simulink library "scarsLibrary"  (R2019b)
settings: Solver=VariableStepAuto  StartTime=0.0  StopTime=10.0  RelTol=1e-3
undefined symbols (not defined in the file): A_x, A_y, A_z, Actuators, added_noise, axis_switch, bb, C_d, decsec, decstart, delay, Detumbling, displacement, Earth, IAU, initDay, initEuler, initYear, linsys1, mag_sat, Magnetorquers, multiplied_noise, Re, rw, scars_library, st_freq, startTime, sun_position, t_power, WGS84
libraries: $bdroot x89, aerolibutil x15, sharedtransform x12, vrlib x9, simulink x6, aerolibtransform2 x2, aerolibgravity2 x2, aerolib6dof2 x2, simulink_extras x2, aerolibatmos2 x1, aerolibnav x1
(part 1 of 2)
settings Model: Creator=asmialek  LastModifiedBy=asmialek

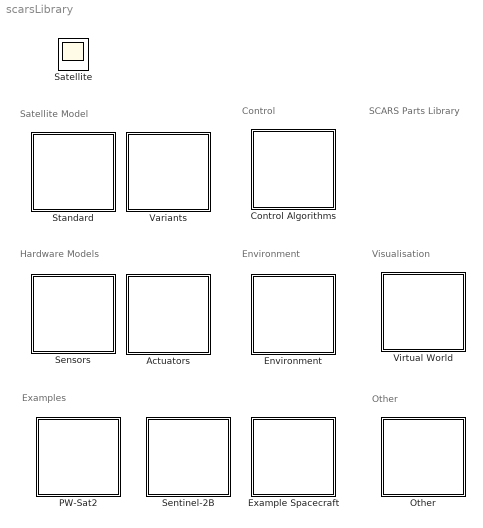
== system scarsLibrary ==
  note: SCARS
      | Parts
      | Library
  note: Environment
  note: Hardware Models
  note: Visualisation
  note: Examples
  note: Control
  note: Satellite Model
  note: Other
  " Control Algorithms " : Subsystem
  Actuators : Subsystem
  Environment : Subsystem
  Example Spacecraft : Subsystem
  Other : Subsystem
  PW-Sat2 : Subsystem
  Sensors : Subsystem
  Sentinel-2B : Subsystem
  Standard : Subsystem
  Variants : Subsystem
  Virtual World : Subsystem
  Satellite : Scope

== system scarsLibrary/ Control Algorithms  ==
  note: Control
  B-dot Algorithm : Subsystem  mask{k_gain=3e-5}
      mask prompts: k_gain "K Gain"
  LQR Controller : Subsystem  mask(Linear-Quadratic Regulator){A=linsys1.A, B=linsys1.B, Q=diag([100 100 100 1 1 1]), R=diag([ 1 1 1 ])}
      mask help: An optimal control method that uses a solution which in simplest form minimizes the quadratic cost function, based on matrices minimizing error in each state and control effor of each input, to generate static gain matrix K.
      mask init:
      | K = lqr(A, B, Q, R)
  Lat/Long to Heading : Subsystem
  PID Controller : Subsystem  mask{Kp=1, Ki=0, Kd=0, pid_sat_max=inf, pid_sat_min=-inf, pid_dz_max=0, pid_dz_min=0}
      mask prompts: Kp "Proportional Gain"; Ki "Integral Gain"; Kd "Derivative Gain"; pid_sat_max "Saturation Max Limit"; pid_sat_min "Saturation Min Limit"; pid_dz_max "Dead Zone Max Limit"; pid_dz_min "Dead Zone Min Limit"

== system scarsLibrary/Actuators ==
  note: Actuators
  Bang-Bang Thrusters : Subsystem
  Basic Thrusters : Subsystem  mask{delay=0, thrust_max=0, thrust_min=0, power=0}
      mask prompts: delay "Transport Delay"; thrust_max "Maximum Thurst"; thrust_min "Minumum Thurst"; power "Power Consumption"
  Drag Sail : Subsystem  mask{area_vector=[0.01 2 2], C_d=[1 1 1], ds_time=0, ds_duration=0, ds_moments=0}
      mask prompts: area_vector "Sail area (X, Y, Z) [m]"; C_d "Drag coefficient (X, Y, Z)"; ds_time "Deployment time [s]"; ds_duration "Deployment duration [s]"; ds_moments "Deployment moments [Nm]"
  Drag Sail (1-axis) : Subsystem  mask{sail_axis_str=X, area=0, C_d=1, deploy_time=0}
      mask prompts: sail_axis_str "Axis perpendicular to sail's plane"; area "Sail area"; C_d "Drag coefficient"; deploy_time "Deployment time"
      mask init:
      | switch sail_axis_str
      |     case 'X'
      |         A_x = area
      |         A_y = 0
      |         A_z = 0
      |     case 'Y'
      |         A_x = 0
      |         A_y = area
      |         A_z = 0
      |     case 'X'
      |         A_x = 0
      |         A_y = 0
      |         A_z = area
      | end
      mask TypeOptions sail_axis_str: X | Y | Z
  Magnetorquer (1-axis) : Subsystem  mask{mag_axis_str=X, L_mt=2.666, R_mt=3.621, l_c_mt=0.25, w_c_mt=7.965e-3, d_w_mt=4.04e-4, mag_vol_max=0, mag_vol_min=0}
      mask prompts: mag_axis_str "Operating Axis"; L_mt "L"; R_mt "R"; l_c_mt "Core Length"; w_c_mt "Core Width"; d_w_mt "Wire Diameter"; mag_vol_max "Max Voltage"; mag_vol_min "Min Voltage"
      mask init:
      | gamma_mt = 2; % empirical constant
      | 
      | mt_pre = gamma_mt*pi*l_c_mt*w_c_mt/(4*d_w_mt);
      | mt_top = (((l_c_mt/w_c_mt)^2)-1)^(3/2);
      | mt_bottom = (l_c_mt/w_c_mt)*acosh(l_c_mt/w_c_mt)-sqrt((l_c_mt/w_c_mt)-1);
      | 
      | mt_gain = mt_pre*((mt_top/mt_bottom)-1);
      | 
      | switch mag_axis_str
      |     case 'X'
      |         axis_switch = 1
      |     case 'Y'
      |         axis_switch = 2
      |     case 'Z'
      |         axis_switch = 3
      | end
      mask TypeOptions mag_axis_str: X | Y | Z
  Magnetorquers : Subsystem  mask{L_mt=2.666, R_mt=3.621, l_c_mt=0.25, w_c_mt=7.965e-3, d_w_mt=4.04e-4, mag_vol_max=3, mag_vol_min=-3}
      mask prompts: L_mt "L"; R_mt "R"; l_c_mt "Core Length"; w_c_mt "Core Width"; d_w_mt "Wire Diameter"; mag_vol_max "Max Voltage"; mag_vol_min "Min Voltage"
      mask init:
      | gamma_mt = 2; % empirical constant
      | 
      | mt_pre = gamma_mt*pi*l_c_mt*w_c_mt/(4*d_w_mt);
      | mt_top = (((l_c_mt/w_c_mt)^2)-1)^(3/2);
      | mt_bottom = (l_c_mt/w_c_mt)*acosh(l_c_mt/w_c_mt)-sqrt((l_c_mt/w_c_mt)-1);
      | 
      | mt_gain = mt_pre*((mt_top/mt_bottom)-1);
  Magnetorquers (Detumbling) : Subsystem  mask{L_mt=2.666, R_mt=3.621, l_c_mt=0.25, w_c_mt=7.965e-3, d_w_mt=4.04e-4, mag_vol_max=0, mag_vol_min=0}
      mask prompts: L_mt "L"; R_mt "R"; l_c_mt "Core Length"; w_c_mt "Core Width"; d_w_mt "Wire Diameter"; mag_vol_max "Max Voltage"; mag_vol_min "Min Voltage"
      mask init: same as scarsLibrary/Actuators/Magnetorquers
  Perfect Actuators : Subsystem  mask{k=1}
      mask prompts: k "Gain"
      mask DialogControl Control2 Prompt: (Add text here)
  Perfect Actuators (1-axis) : Subsystem  mask{axis_switch=X, k=1}
      mask prompts: axis_switch "Operating Axis"; k "Gain"
      mask TypeOptions axis_switch: X | Y | Z
      mask DialogControl Control2 Prompt: (Add text here)
  "Perfect Actuators (1-axis, vector)" : Subsystem  mask{axis_switch=X, k=1}
      mask prompts: axis_switch "Operating Axis"; k "Gain"
      mask TypeOptions axis_switch: X | Y | Z
      mask DialogControl Control2 Prompt: (Add text here)
  "Reaction Wheel (1-axis, X/Y/Z)" : Subsystem  mask{axis_switch=X, N=25e-3, R=0.1, J=1, c=0.0001, vel_max=0.0001, torq_max=0, i_max=0, rw_power=0.0001, rw_freq=0.1}
      mask prompts: axis_switch "Operating Axis"; N "Torque per unit current [Nm]"; R "Armature restitance [Ohm]"; J "Moment of inertia of wheel plus motor [kgm2]"; c "Viscous friction coefficient"; vel_max "Maximum angular velocity [rad/s]"; torq_max "Maximum torque [Nm]"; i_max "Maximum current [A]"; rw_power "Output Noise Power"; rw_freq "Noise Frequency"
      mask TypeOptions axis_switch: X | Y | Z
  "Reaction Wheel (1-axis, vector)" : Subsystem  mask(Reaction Wheel){op_vect=[1 1 1], N=(1.5e-3)/0.5, R=12, J=300e-3, c=0.0001, vel_max=6000*2*pi/60, torq_max=1.5e-3, i_max=0.5, rw_power=0.0001, rw_freq=0.1}
      mask prompts: op_vect "Operating Axis (X,Y,Z)"; N "Torque per unit current [Nm]"; R "Armature restitance [Ohm]"; J "Moment of inertia of wheel plus motor [kgm2]"; c "Viscous friction coefficient"; vel_max "Maximum angular velocity [rad/s]"; torq_max "Maximum torque [Nm]"; i_max "Maximum current [A]"; rw_power "Output Noise Power"; rw_freq "Noise Frequency"
      mask help:
      | Fast attitude control can be also achieved by the use of reaction wheels - mechanisms consisting of rotating flywheel and proportional electromagnetic torquer, such as DC motor. This allows for very precise attitude maneuvers, with the possibility to eliminate most disturbance torques.
      |
      | Inputs:
      |  Cmd - Reaction Wheel commadn voltage [V]
      |  SatStates - Bus signal from Satellite  Dynamics
      |
      | Outputs:
      |  Moment - Torque that is produced by the wheel and which acts on spacecraft (in Body frame) [Nm]
      |  WheelVel - Angular velocity of the wheel [rad/s]
      mask init:
      | op_vect = op_vect/norm(op_vect);
  Reaction Wheels : Subsystem
  Thruster : Subsystem

== system scarsLibrary/Environment ==
  Atmosphere [kg/m^3] : Subsystem
  Atmospheric Drag [N] : Subsystem
  Drag [N] : Subsystem
  Environment : Subsystem
  Gravity [N] : Subsystem  mask(Gravity){mass=0}
      mask prompts: mass "Object mass [kg]"
      mask help: Main centripetal force acting on a spacecraft on any orbit is gravity, derived from Newton's law of universal gravitation.
  Magnetic Field [nT] : Subsystem
  Sun's Position [km] : Subsystem

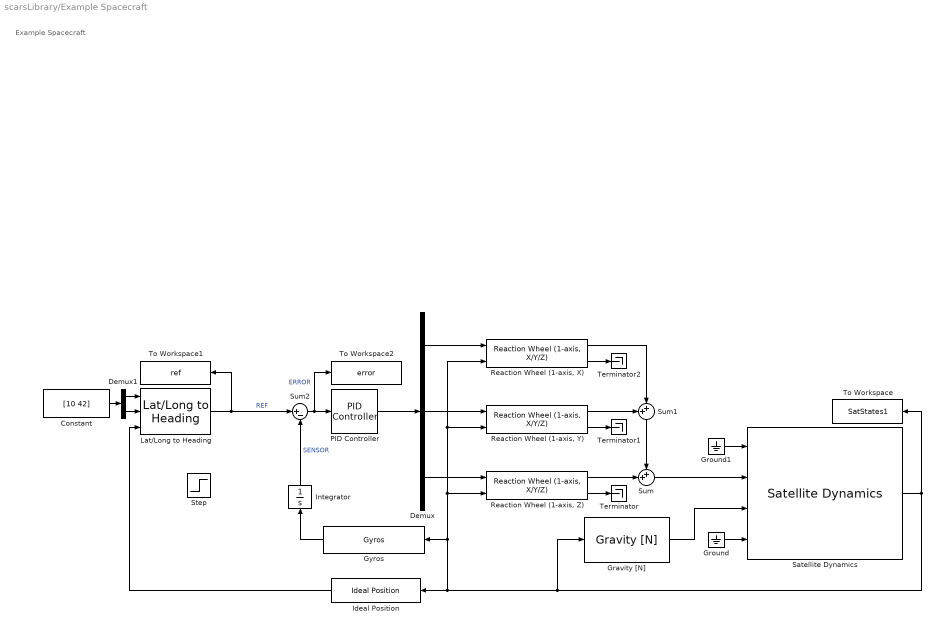
== system scarsLibrary/Example Spacecraft ==
  note: Example Spacecraft
  Constant : Constant  Value=[10 42]
  Demux : Demux  Outputs=3
  Demux1 : Demux  Outputs=2
  Gravity [N] : $bdroot/Environment/Gravity [N]  mass=1
  Ground : Ground
  Ground1 : Ground
  Gyros : $bdroot/Sensors/Gyros  g_wn=14500  g_zeta=sqrt(2)/2  g_freq=10  g_bias=0  g_power=(2*pi*0.04/360)^2  g_max=deg2rad(75)  g_min=-deg2rad(75)
  Ideal Position : $bdroot/Sensors/Ideal Position  SystemSampleTime=-1  Latency=0  AutoFrameSizeCalculation=off
  Integrator : Integrator  InitialCondition=[0.76 2.32 1.71]
  Lat/Long to Heading : $bdroot/ Control Algorithms /Lat//Long to Heading  SystemSampleTime=-1  Latency=0  AutoFrameSizeCalculation=off
  PID Controller : $bdroot/ Control Algorithms /PID Controller  Kp=700  Ki=0.01  Kd=1000  pid_sat_max=inf  pid_sat_min=-inf  pid_dz_max=0  pid_dz_min=0
  "Reaction Wheel (1-axis, X)" : $bdroot/Actuators/Reaction Wheel (1-axis, X//Y//Z)  axis_switch=X  N=(1.5e-3)/0.5  R=12  J=300e-3  c=0  vel_max=6000*2*pi/60  torq_max=1.5e-3  i_max=0.5  rw_power=0  rw_freq=0.1
  "Reaction Wheel (1-axis, Y)" : $bdroot/Actuators/Reaction Wheel (1-axis, X//Y//Z)  axis_switch=Y  N=(1.5e-3)/0.5  R=12  J=300e-3  c=0  vel_max=6000*2*pi/60  torq_max=1.5e-3  i_max=0.5  rw_power=0  rw_freq=0.1
  "Reaction Wheel (1-axis, Z)" : $bdroot/Actuators/Reaction Wheel (1-axis, X//Y//Z)  axis_switch=Z  N=(1.5e-3)/0.5  R=12  J=300e-3  c=0  vel_max=6000*2*pi/60  torq_max=1.5e-3  i_max=0.5  rw_power=0  rw_freq=0.1
  Satellite Dynamics : $bdroot/Standard/Satellite Dynamics  Parameter4=Keplerian Elements  epoch=0  mass=0  a=6356e3+400e3  e=0  incl=0  RA=0  w=0  TA=0  initEuler=[0 0 0]  initEulerRates=[0 0 0]  TA_copy=0  TA_copy_copy=400e3  TA_copy_copy_copy=[10 25]  TA_copy_copy_copy_copy=[10 25]  initEuler_copy=[0 0 0]  initEulerRates_copy=[0 0 0]
  Step : Step  Time=180  SampleTime=0
  Sum : Sum  Inputs=++|
  Sum1 : Sum  Inputs=++|
  Sum2 : Sum  Inputs=|+-
  Terminator : Terminator
  Terminator1 : Terminator
  Terminator2 : Terminator
  To Workspace : ToWorkspace  VariableName=SatStates1  SaveFormat=Timeseries  SampleTime=-1
  To Workspace1 : ToWorkspace  VariableName=ref  SaveFormat=Timeseries  SampleTime=-1
  To Workspace2 : ToWorkspace  VariableName=error  SaveFormat=Timeseries  SampleTime=-1
  wires:
  Ground/1 -> Satellite Dynamics/4
  Integrator/1 -> Sum2/2  "SENSOR"
  Demux1/1 -> Lat/Long to Heading/1
  Demux1/2 -> Lat/Long to Heading/2
  Demux/2 -> "Reaction Wheel (1-axis, Y)"/1
  PID Controller/1 -> Demux/1
  "Reaction Wheel (1-axis, Y)"/1 -> Sum1/1
  Demux/3 -> "Reaction Wheel (1-axis, Z)"/1
  "Reaction Wheel (1-axis, Y)"/2 -> Terminator1/1
  "Reaction Wheel (1-axis, X)"/1 -> Sum1/2
  "Reaction Wheel (1-axis, X)"/2 -> Terminator2/1
  "Reaction Wheel (1-axis, Z)"/2 -> Terminator/1
  Gyros/1 -> Integrator/1
  "Reaction Wheel (1-axis, Z)"/1 -> Sum/2
  Demux/1 -> "Reaction Wheel (1-axis, X)"/1
  Sum2/1 -> To Workspace2/1, PID Controller/1  "ERROR"
  Constant/1 -> Demux1/1
  Ideal Position/1 -> Lat/Long to Heading/3
  Sum1/1 -> Sum/1
  Gravity [N]/1 -> Satellite Dynamics/3
  Sum/1 -> Satellite Dynamics/2
  Ground1/1 -> Satellite Dynamics/1
  Satellite Dynamics/1 -> Ideal Position/1, Gyros/1, "Reaction Wheel (1-axis, X)"/2, "Reaction Wheel (1-axis, Y)"/2, "Reaction Wheel (1-axis, Z)"/2, Gravity [N]/1, To Workspace/1
  Lat/Long to Heading/1 -> Sum2/1, To Workspace1/1  "REF"

== system scarsLibrary/Other ==
  note: Other
  Actuator Noise : Subsystem
  Scope : Scope  NumInputPorts=2
  Subsystem : Subsystem
  Subsystem1 : Subsystem
  Subsystem4 : Subsystem
  Unit Pulse : Subsystem
  Unit Pulse Product : Subsystem
  Vector Norm : Subsystem
  "Vector Single to 3D " : Subsystem  mask{axis_switch=axis_switch}
  wires:
  Subsystem1/2(<X_ECEF>) -> Scope/2
  Subsystem1/1(<V_ECEF>) -> Scope/1

== system scarsLibrary/PW-Sat2 ==
  note: PW-Sat2
  Bus Selector : BusSelector  OutputSignals=lla,X_ECEF,V_B,A_B,Euler_B,Omega_B
  Drag Sail : Subsystem  AncestorBlock=scars_library/Actuators/Drag Sail  mask(Drag Sail){area_vector=[4 0 0], C_d=[1 0 0], ds_time=25.3*24*60*60, ds_duration=100, ds_moments=[1e-5 1e-5 1e-5]}
      mask prompts: area_vector "Sail area (X, Y, Z) [m]"; C_d "Drag coefficient (X, Y, Z)"; ds_time "Deployment time [s]"; ds_duration "Deployment duration [s]"; ds_moments "Deployment moments [Nm]"
      mask help: Drag sails use the occurrence of partial atmosphere to lower satellite's tangential velocity and therefore to quicken the deorbitation of the spacecraft. The premise is to increase area-to-mass-ratio by deploying a large and lightweight structure near the planned end-of-life of the spacecraft.
  Environment : Subsystem  AncestorBlock=scars_library/Environment/Environment  mask{area_vector=[0 0 0]}
      mask prompts: area_vector "Area Vector"
  Magnetorquers (Detumbling) : Subsystem  AncestorBlock=scars_library/Actuators/Magnetorquers (Detumbling)  mask(Magnetorquers){k_gain=-0.1, Parameter11=3, L_mt=2.666, R_mt=3.621, l_c_mt=0.25, w_c_mt=7.965e-3, d_w_mt=4.04e-4, mag_vol_max=5, Parameter9=0.2}
      mask prompts: k_gain "B-Dot algorithm gain"; Parameter11 "Maximum actuation error"; L_mt "Circuit inductance"; R_mt "Circuit resistance"; l_c_mt "Core length"; w_c_mt "Core width"; d_w_mt "Wire diameter"; mag_vol_max "Max voltage"; Parameter9 "Nominal magnetic dipole [Am^2]"
      mask help: A magnetorquer is an attitude actuator which uses Earth's geomagnetic field to generate controlling torque. The active part in the magnetorquer is the solenoid, which generates the magnetic dipole moment proportional to the current conducted by the coil.
      mask init: same as scarsLibrary/Actuators/Magnetorquers
  Satellite Dynamics : Subsystem  AncestorBlock=scars_library/Advanced/Satellite Dynamics
      mask Display: image('pw-sat-2__2.jpg'); % Use "Edit Image" on toolstrip to change.
  Scope : Scope  NumInputPorts=6
  Selector : Selector  InputPortWidth=3  IndexOptions=Index vector (dialog)  Indices=3  OutputSizes=1
  Sum : Sum  Inputs=+|+|
  To Workspace : ToWorkspace  VariableName=SatStates  SaveFormat=Timeseries  SampleTime=-1
  wires:
  Sum/1 -> Satellite Dynamics/2(M_sat)
  Bus Selector/3 -> Scope/3  "<V_B>"
  Bus Selector/6 -> Scope/6  "<Omega_B>"
  Environment/3(Moments) -> Satellite Dynamics/4(M_env)
  Satellite Dynamics/1(SatStates) -> Bus Selector/1, Magnetorquers (Detumbling)/2(SatStates), Drag Sail/1(SatStates), Environment/1(SatStates), To Workspace/1
  Bus Selector/4 -> Scope/4  "<A_B>"
  Drag Sail/2(Moment) -> Sum/1
  Bus Selector/2 -> Scope/2  "<X_ECEF>"
  Environment/1(Env) -> Drag Sail/2(Env), Magnetorquers (Detumbling)/1(Env)
  Environment/2(Forces) -> Satellite Dynamics/3(F_env)
  Drag Sail/1(Force) -> Satellite Dynamics/1(F_sat)
  Magnetorquers (Detumbling)/1(Torque) -> Sum/2
  Bus Selector/5 -> Scope/5  "<Euler_B>"
  Selector/1 -> Scope/1
  Bus Selector/1 -> Selector/1  "<lla>"

== system scarsLibrary/Sensors ==
  note: Sensors
  Accelerometer : Subsystem  mask{acc=[0 0 0], w_a=190, z_a=0.707, a_bias=[0 0 0], a_pow=0.001, a_max=inf, a_min=-inf, freq=0}
      mask prompts: acc "Sensor Location"; w_a "Natural Frequency"; z_a "Damping Ratio"; a_bias "Measurement Bias"; a_pow "Noise Power"; a_max "Upper Output Limit"; a_min "Lower Output Limit"; freq "Sampling Frequency [Hz]"
  Earth- & Sun-sensor : Subsystem
  GPS Receiver : Subsystem
  Gyros : Subsystem  mask{g_wn=1000*2*pi, g_zeta=sqrt(2)/2, g_freq=80, g_bias=0, g_power=(0.04)^2, g_max=deg2rad(100), g_min=-deg2rad(100)}
      mask prompts: g_wn "Natural Frequency [Hz]"; g_zeta "Damping Ratio"; g_freq "Operating Frequency [Hz]"; g_bias "Measurement Bias [rad/s]"; g_power "Noise Power (RND^2)"; g_max "Upper Output Limit [rad/s]"; g_min "Lower Output Limit [rad/s]"
      mask init:
      | g_wn = g_wn*2*pi;
  Ideal Angle : Subsystem
  Ideal Position : Subsystem
  Ideal Rate : Subsystem
  Magnetometer : Subsystem  mask{m_power=0.1, m_freq=10, m_bias=[0.01 0.01 0.01]}
      mask prompts: m_power "Noise Power Spectral Density"; m_freq "Sampling Frequncy [Hz]"; m_bias "Measurement Bias [nT]"
  Simple Angle : Subsystem
  Simple Position : Subsystem
  Simple Rate : Subsystem
  Star Tracker : Subsystem  mask{st_vector=[0 0 -1], st_ex_sun=20, st_ex_earth=20, st_lost=5, Parameter5=10}
      mask prompts: st_vector "Poiting Vector with respect to Body Axes"; st_ex_sun "Sun Exclusive Angle [deg]"; st_ex_earth "Earth Exclusive Angle [deg]"; st_lost "Average Lost Space Solving Time [s]"; Parameter5 "Update Rate [Hz]"

== system scarsLibrary/Sentinel-2B ==
  note: Sentinel-2B
  Actuators : Subsystem
  Environment : $bdroot/Environment/Environment  SystemSampleTime=-1  Latency=0  AutoFrameSizeCalculation=off
  OBC : Subsystem
  Satellite Dynamics : $bdroot/Standard/Satellite Dynamics  Parameter4=Keplerian Elements  epoch=0  mass=0  a=6356e3+400e3  e=0  incl=0  RA=0  w=0  TA=0  initEuler=[0 0 0]  initEulerRates=[0 0 0]  TA_copy=0  TA_copy_copy=400e3  TA_copy_copy_copy=[10 25]  TA_copy_copy_copy_copy=[10 25]  initEuler_copy=[0 0 0]  initEulerRates_copy=[0 0 0]  mask(Sattellite Dynamics){}
      mask Display: image('C:\master_thesis\scars_toolbox\resources\sentinel.jpg'); % Use "Edit Image" on toolstrip to change.
  Sensors : Subsystem
  wires:
  Sensors/1(Sensors) -> OBC/1(Sensors)
  OBC/3(MTQ) -> Actuators/4(MTQ)
  Environment/3 -> Sensors/2("Env "), Actuators/5(Env)
  Satellite Dynamics/1 -> Environment/1, Sensors/1("SatStates "), Actuators/1(SatStates)
  Actuators/2(Force) -> Satellite Dynamics/2
  Environment/1 -> Satellite Dynamics/3
  Environment/2 -> Satellite Dynamics/4
  OBC/1(RW) -> Actuators/2(RW)
  Actuators/1(Moment) -> Satellite Dynamics/1
  OBC/2(THR) -> Actuators/3(THR)

== system scarsLibrary/Standard ==
  Satellite Dynamics : Subsystem  mask(Sattellite Dynamics){Parameter4=Keplerian Elements, epoch=0, mass=0, a=6356e3+400e3, e=0, incl=0, RA=0, w=0, TA=0, initEuler=[0 0 0], initEulerRates=[0 0 0], TA_copy=0, TA_copy_copy=400e3, TA_copy_copy_copy=[10 25], TA_copy_copy_copy_copy=[10 25], initEuler_copy=[0 0 0], initEulerRates_copy=[0 0 0]}
      mask prompts: Parameter4 "Initialization method"; epoch "Epoch of ECI frame"; mass "Satellite mass [kg]"; a "Semi-major axis [m]"; e "Eccentricity"; incl "Inclination [deg]"; RA "Right ascension of the ascending node [deg]"; w "Argument of periapsis [deg]"; TA "True anomaly [deg]"; initEuler "Initial Euler orientation with reference to NED [deg]"; initEulerRates "Initial body roation rates [deg/s]"; TA_copy "True anomaly [deg]"; TA_copy_copy "Altitude [m]"; TA_copy_copy_copy "Geodetic position (latitude, longitude) [deg]"; TA_copy_copy_copy_copy "Body velocity in NED frame [m/s]"; initEuler_copy "Euler orientation with reference to NED [deg]"; initEulerRates_copy "Body roation rates [deg/s]"
      mask help: Main block of SCARS Toolbox. Allows for setting up satellite dynamics in with initial values in various coordinate system. The order of all axis, in position, velocity, orientation and rates, is always XYZ, unless otherwise stated.
      mask init:
      | Re = 6356e3;
      | G = 6.6743015e-11;
      | Re = 6356e3;
      | Me = 5.972e24;
      | 
      | if incl == 0
      |     incl = 0.00000001
      | end
      | 
      | mu = 3.986004418e14;
      | 
      | initYear = 2000;
      | initDay = 0;
      | utc = [2000 1 1 12 0 0];
      | julian = juliandate(utc);
      | juliansec = juliandate([2000 1 1 12 0 1]) - juliandate([2000 1 1 12 0 0]);
      | decstart = decyear(utc);
      | decsec = decyear(2000,1,1,12,0,1) - decyear(2000,1,1,12,0,0);
      | [r_eci, v_eci] = kep2eci(a, e, deg2rad(RA), deg2rad(incl), deg2rad(w), deg2rad(TA), mu)
      | [r_ecef,v_ecef] = eci2ecef(utc,r_eci,v_eci) % this is from aerorpace tb
      | r_lla = ecef2lla(r_ecef') % this too
      | assignin('base','R_LLA', r_lla)
      | r_lla(1:2)
      mask TypeOptions Parameter4: Keplerian Elements | ECEF Position, Velocity, Rotation | LLA Position & NED Velocity, Rotation
      mask DialogControl Container7_copy_copy Prompt: Keplerian Elements
      mask DialogControl Container7_copy Prompt: ECEF Pos, Vel, Rot
      mask DialogControl Container7 Prompt: LLA Pos & NED Vel, Rot

== system scarsLibrary/Variants ==
  Subsystem : Subsystem
  Subsystem1 : Subsystem
  Subsystem2 : Subsystem
  Subsystem3 : Subsystem

== system scarsLibrary/Virtual World ==
  note: Visualisation
  Position to VRML : Subsystem
  Quaternion to VRML : Subsystem
  SCARS VR Sink : vrlib/VR Sink  InstantiateOnLoad=on  SampleTime=-1  ViewEnable=on  RemoteChange=off  RemoteView=off  FieldsWritten=Sat.rotation.4.1.1.double#Sat.translation.3.1.1.double#Sun.translation.3.1.1.double  WorldFileName=sat_test.wrl  AutoView=off  VideoDimensions=[]  AllowVariableSize=off  FigureProperties="{'Position', 'Name', 'Viewpoint', 'CameraBound', 'CameraDirection', 'CameraPosition', 'CameraUpVector', 'ZoomFactor', 'Antialiasing', 'Headlight', 'Lighting', 'NavPanel', 'Sound', 'StatusBar', 'Stereo3D', 'Stereo3DCameraOffset', 'Stereo3DHIT', 'ToolBar', 'Textures', 'Transparency', 'Triad', 'Wireframe', 'NavZones', 'NavMode', 'NavSpeed', 'CaptureFileFormat', 'CaptureFileName', 'Record2DCompressMethod', 'Record2DCompressQuality', 'Record2D', 'Record2DFileName', 'Record2DFPS'; [5.0000000000000000e+00   9.2000000000000000e+01   5.7600000000000000e+02   3.5000000000000000e+02], '', 'Sat Cam', 'on', [0.0000000000000000e+00   0.0000000000000000e+00  -1.0000000000000000e+00], [0.0000000000000000e+00   0.0000000000000000e+00   0.0000000000000000e+00], [0.0000000000000000e+00   1.0000000000000000e+00   0.0000000000000000e+00], [1.0000000000000000e+00], 'on', 'on', 'on', 'halfbar', 'on', 'on', 'off', [1.0000000149011612e-01], [0.0000000000000000e+00], 'on', 'on', 'on', 'none', 'off', 'off', 'fly', 'normal', 'tif', '%f_anim_%n.tif', 'auto', [7.5000000000000000e+01], 'off', '%f_anim_%n.avi', 'auto'}"
      settings: SourceProductName=Simulink
  SCARS to VRML : Subsystem
  Sun's Position to ECEF : Subsystem
  wires:
  SCARS to VRML/2(Sat Pos) -> SCARS VR Sink/2
  SCARS to VRML/3(Sun Pos) -> SCARS VR Sink/3
  SCARS to VRML/1(Sat Rot) -> SCARS VR Sink/1

== system scarsLibrary/ Control Algorithms /B-dot Algorithm ==
  B : Inport
  Derivative : Derivative
  Divide : Product  Inputs=*/
  Gain2 : Gain  Gain=k_gain
  Square : Math  Operator=square  SignedPower=off  SaturateOnIntegerOverflow=on
  Vector Norm : $bdroot/Vector Norm  SystemSampleTime=-1  Latency=0  AutoFrameSizeCalculation=off
  m_ctrl : Outport
  wires:
  Derivative/1 -> Gain2/1
  Vector Norm/1 -> Square/1
  Square/1 -> Divide/2
  Divide/1 -> m_ctrl/1  "ref"
  Gain2/1 -> Divide/1
  B/1 -> Vector Norm/1, Derivative/1

== system scarsLibrary/ Control Algorithms /LQR Controller ==
  x : Inport
  Gain : Gain  Gain=-K  Multiplication=Matrix(K*u)
  u : Outport
  wires:
  x/1 -> Gain/1
  Gain/1 -> u/1

== system scarsLibrary/ Control Algorithms /Lat//Long to Heading ==
  Latitude : Inport
  Longitude : Inport  Port=2
  X_ECEF : Inport  Port=3
  Constant : Constant  Value=0
  LLA to ECEF Position : aerolibtransform2/LLA to ECEF Position  units=Metric (MKS)  ptype=Earth (WGS84)  F=1/298.257223563  R=6378137
      settings: SourceProductName=Aerospace Blockset  SourceProductBaseCode=AE
  Mux : Mux  Inputs=2
  Subsystem : $bdroot/Subsystem  SystemSampleTime=-1  Latency=0  AutoFrameSizeCalculation=off
  Sum : Sum  Inputs=-|+
  Euler_B : Outport
  wires:
  Constant/1 -> LLA to ECEF Position/2
  Latitude/1 -> Mux/1
  Longitude/1 -> Mux/2
  Mux/1 -> LLA to ECEF Position/1
  LLA to ECEF Position/1 -> Sum/1
  X_ECEF/1 -> Sum/2
  Sum/1 -> Subsystem/1
  Subsystem/1 -> Euler_B/1

== system scarsLibrary/ Control Algorithms /PID Controller ==
  Error : Inport
  Constant : Constant  Value=0
  Constant1 : Constant  Value=0
  Derivative : Derivative
  Gain : Gain  Gain=-1
  Integrator2 : Integrator  ExternalReset=either
  Kd : Gain  Gain=Kd
  Ki : Gain  Gain=Ki
  Kp : Gain  Gain=Kp
  Saturation : Saturate  UpperLimit=0.1  LowerLimit=-0.1
  Sum4 : Sum  Inputs=+++
  Switch : Switch  Criteria=u2 > Threshold  Threshold=pid_dz_max
  Switch1 : Switch  Threshold=pid_dz_max
  Switch2 : Switch  Criteria=u2 > Threshold  Threshold=-pid_dz_min
  Out : Outport
  wires:
  Integrator2/1 -> Ki/1  "theta"
  Sum4/1 -> Out/1
  Kp/1 -> Sum4/1
  Ki/1 -> Saturation/1
  Derivative/1 -> Kd/1
  Kd/1 -> Sum4/3
  Saturation/1 -> Sum4/2
  Switch1/1 -> Derivative/1, Kp/1, Integrator2/1
  Switch/1 -> Switch1/1
  Constant/1 -> Switch/3
  Constant1/1 -> Switch2/3
  Gain/1 -> Switch2/2
  Error/1 -> Integrator2/2, Switch/1, Switch/2, Gain/1, Switch2/1, Switch1/2
  Switch2/1 -> Switch1/3

== system scarsLibrary/Actuators/Bang-Bang Thrusters ==
  TorqueCmd : Inport
  Constant : Constant  Value=displacement
  Demux : Demux  Outputs=3
  Gain : Gain  Gain=-1
  Mux : Mux  Inputs=3
  Product : Product
  Thruster Pitch : Subsystem
  Thruster Roll : Subsystem
  Thruster Yaw : Subsystem
  Torque : Outport  VectorParamsAs1DForOutWhenUnconnected=off
  Moments : Outport  Port=2  VectorParamsAs1DForOutWhenUnconnected=off
  wires:
  Gain/1 -> Product/1, Torque/1
  Mux/1 -> Gain/1
  Demux/3 -> Thruster Yaw/1(Torque)
  Demux/1 -> Thruster Roll/1(Torque)
  Demux/2 -> Thruster Pitch/1(Torque)
  TorqueCmd/1 -> Demux/1
  Thruster Yaw/1(Torque Out) -> Mux/3
  Thruster Pitch/1(Torque Out) -> Mux/2
  Thruster Roll/1(Torque Out) -> Mux/1
  Constant/1 -> Product/2
  Product/1 -> Moments/1

== system scarsLibrary/Actuators/Basic Thrusters ==
  ActuatorCmd : Inport
  Abs : Abs
  Constant : Constant  Value=t_power
  Product : Product
  Saturation : Saturate  UpperLimit=thrust_max  LowerLimit=thrust_min
  Sign : Signum
  Transport Delay : TransportDelay  DelayTime=delay
  Force : Outport
  Power : Outport  Port=2
  wires:
  Abs/1 -> Saturation/1
  Sign/1 -> Product/2
  Saturation/1 -> Product/1
  Product/1 -> Force/1
  Transport Delay/1 -> Sign/1, Abs/1
  Constant/1 -> Power/1
  ActuatorCmd/1 -> Transport Delay/1

== system scarsLibrary/Actuators/Drag Sail ==
  SatStates : Inport
  Density : Inport  Port=2
  Add : Sum
  Deployment Duration : Step  Time=ds_time+ds_duration  After=-1  SampleTime=0
  Deployment Time : Step  Time=ds_time  SampleTime=0
  Depoloyment Moments : Constant  Value=ds_moments
  "Drag " : Subsystem
  Gain : Gain
  Product : Product
  Product1 : Product
  Product3 : Product
  Force : Outport
  Moment : Outport  Port=2
  wires:
  Density/1 -> "Drag "/2(Density)
  Product/1 -> Gain/1
  SatStates/1 -> "Drag "/1(SatStates)
  Deployment Time/1 -> Product1/1, Product/2
  "Drag "/1(Force) -> Product/1
  Add/1 -> Moment/1
  Depoloyment Moments/1 -> Product1/2, Product3/1
  Deployment Duration/1 -> Product3/2
  Product1/1 -> Add/1
  Product3/1 -> Add/2
  Gain/1 -> Force/1

== system scarsLibrary/Actuators/Drag Sail (1-axis) ==
  SatStates : Inport
  Bus Element In2 : Inport  Port=2  PortName=Env  Element=rho
  "Drag " : Subsystem
  Product : Product
  Step : Step  Time=5*24*60*60  SampleTime=0
  Force : Outport
  wires:
  "Drag "/1(Force) -> Product/1
  Step/1 -> Product/2
  SatStates/1 -> "Drag "/1(SatStates)
  Product/1 -> Force/1
  Bus Element In2/1 -> "Drag "/2(Density)

== system scarsLibrary/Actuators/Magnetorquer (1-axis) ==
  Voltage : Inport
  Bus Element In : Inport  Port=2  PortName=Env  Element=Magnetic Field [nT]
  Bus Element In1 : Inport  Port=3  PortName=SatStates  Element=NED2Body
  " Coil Gain" : Gain  Gain=mt_gain
  Circuit Transfer Fcn : TransferFcn  Denominator=[L_mt R_mt]
  Cross Product : vrlib/Utilities/Cross Product
      settings: SourceProductName=Simulink
  Direction Cosine Matrix to Quaternions : sharedtransform/Direction Cosine Matrix  to Quaternions  aMode=0  action=None  tolerance=eps(2)
      settings: SourceProductName=Aerospace Blockset  SourceProductBaseCode=AE
  Gain1 : Gain  Gain=1e-9
  Quaternion Rotation : aerolibutil/Quaternion Rotation
  Saturation : Saturate  UpperLimit=mag_sat  LowerLimit=-mag_sat
  "Vector Single to 3D " : $bdroot/Actuators/Vector Single to 3D   axis_switch=axis_switch
  Torque : Outport
  wires:
  Gain1/1 -> Quaternion Rotation/2
  Circuit Transfer Fcn/1 -> " Coil Gain"/1
  Saturation/1 -> Circuit Transfer Fcn/1
  Bus Element In/1 -> Gain1/1
  Quaternion Rotation/1 -> Cross Product/2
  Bus Element In1/1 -> Direction Cosine Matrix to Quaternions/1
  Direction Cosine Matrix to Quaternions/1 -> Quaternion Rotation/1
  Cross Product/1 -> Torque/1
  " Coil Gain"/1 -> "Vector Single to 3D "/1
  Voltage/1 -> Saturation/1
  "Vector Single to 3D "/1 -> Cross Product/1

== system scarsLibrary/Actuators/Magnetorquers ==
  Voltage : Inport
  Bus Element In : Inport  Port=2  PortName=Env  Element=Magnetic Field [nT]
  Bus Element In1 : Inport  Port=3  PortName=SatStates  Element=DCM_NED2B
  Cross Product : vrlib/Utilities/Cross Product
      settings: SourceProductName=Simulink
  Demux : Demux  Outputs=3
  Direction Cosine Matrix to Quaternions : sharedtransform/Direction Cosine Matrix  to Quaternions  aMode=0  action=None  tolerance=eps(2)
      settings: SourceProductName=Aerospace Blockset  SourceProductBaseCode=AE
  Gain : Gain  Gain=mt_gain
  Gain1 : Gain  Gain=1e-9
  Mux : Mux  Inputs=3
  Quaternion Rotation : aerolibutil/Quaternion Rotation
  Saturation : Saturate  UpperLimit=mag_sat  LowerLimit=-mag_sat
  Transfer Fcn : TransferFcn  Denominator=[L_mt R_mt]
  Transfer Fcn1 : TransferFcn  Denominator=[L_mt R_mt]
  Transfer Fcn2 : TransferFcn  Denominator=[L_mt R_mt]
  Moment : Outport
  wires:
  Gain1/1 -> Quaternion Rotation/2
  Mux/1 -> Gain/1
  Transfer Fcn/1 -> Mux/1
  Transfer Fcn1/1 -> Mux/3
  Transfer Fcn2/1 -> Mux/2
  Demux/1 -> Transfer Fcn/1
  Demux/2 -> Transfer Fcn2/1
  Demux/3 -> Transfer Fcn1/1
  Saturation/1 -> Demux/1
  Bus Element In/1 -> Gain1/1
  Quaternion Rotation/1 -> Cross Product/2
  Bus Element In1/1 -> Direction Cosine Matrix to Quaternions/1
  Direction Cosine Matrix to Quaternions/1 -> Quaternion Rotation/1
  Cross Product/1 -> Moment/1
  Gain/1 -> Cross Product/1
  Voltage/1 -> Saturation/1

== system scarsLibrary/Actuators/Magnetorquers (Detumbling) ==
  Bus Element In : Inport  PortName=Env  Element=Magnetic Field [nT]
  Bus Element In1 : Inport  Port=2  PortName=SatStates  Element=DCM_NED2B
  B-dot Algorithm : $bdroot/ Control Algorithms /B-dot Algorithm  k_gain=3e-5
  Cross Product : vrlib/Utilities/Cross Product
      settings: SourceProductName=Simulink
  Demux : Demux  Outputs=3
  Direction Cosine Matrix to Quaternions : sharedtransform/Direction Cosine Matrix  to Quaternions  aMode=0  action=None  tolerance=eps(2)
      settings: SourceProductName=Aerospace Blockset  SourceProductBaseCode=AE
  Gain : Gain  Gain=mt_gain
  Gain1 : Gain  Gain=1e-9
  Mux : Mux  Inputs=3
  PID Controller : $bdroot/ Control Algorithms /PID Controller  Kp=1  Ki=0  Kd=0  pid_sat_max=inf  pid_sat_min=-inf  pid_dz_max=0  pid_dz_min=0
  Quaternion Rotation : aerolibutil/Quaternion Rotation
  Saturation : Saturate  UpperLimit=mag_sat  LowerLimit=-mag_sat
  Sum : Sum  Inputs=-+|
  Transfer Fcn : TransferFcn  Denominator=[L_mt R_mt]
  Transfer Fcn1 : TransferFcn  Denominator=[L_mt R_mt]
  Transfer Fcn2 : TransferFcn  Denominator=[L_mt R_mt]
  Torque : Outport
  wires:
  PID Controller/1 -> Saturation/1
  Demux/3 -> Transfer Fcn1/1
  B-dot Algorithm/1 -> Sum/2
  Demux/1 -> Transfer Fcn/1
  Saturation/1 -> Demux/1
  Sum/1 -> PID Controller/1
  Direction Cosine Matrix to Quaternions/1 -> Quaternion Rotation/1
  Quaternion Rotation/1 -> Cross Product/2, B-dot Algorithm/1
  Mux/1 -> Gain/1
  Demux/2 -> Transfer Fcn2/1
  Transfer Fcn/1 -> Mux/1
  Bus Element In/1 -> Gain1/1
  Transfer Fcn1/1 -> Mux/3
  Cross Product/1 -> Torque/1
  Transfer Fcn2/1 -> Mux/2
  Bus Element In1/1 -> Direction Cosine Matrix to Quaternions/1
  Gain/1 -> Sum/1, Cross Product/1  "m"
  Gain1/1 -> Quaternion Rotation/2

== system scarsLibrary/Actuators/Perfect Actuators ==
  ActuatorCmd : Inport
  Demux : Demux  Outputs=3
  Gain : Gain
  Mux : Mux  Inputs=3
  Out : Outport
  wires:
  Demux/3 -> Mux/3
  Mux/1 -> Gain/1
  Demux/1 -> Mux/1
  ActuatorCmd/1 -> Demux/1
  Demux/2 -> Mux/2
  Gain/1 -> Out/1

== system scarsLibrary/Actuators/Perfect Actuators (1-axis) ==
  ActuatorCmd : Inport
  Gain : Gain
  "Vector Single to 3D  " : $bdroot/Actuators/Vector Single to 3D   axis_switch=axis_switch
  Out : Outport
  wires:
  Gain/1 -> "Vector Single to 3D  "/1
  ActuatorCmd/1 -> Gain/1
  "Vector Single to 3D  "/1 -> Out/1

== system scarsLibrary/Actuators/Perfect Actuators (1-axis, vector) ==
  ActuatorCmd : Inport
  Gain : Gain
  "Vector Single to 3D  " : $bdroot/Actuators/Vector Single to 3D   axis_switch=axis_switch
  Out : Outport
  wires:
  "Vector Single to 3D  "/1 -> Out/1
  ActuatorCmd/1 -> Gain/1
  Gain/1 -> "Vector Single to 3D  "/1

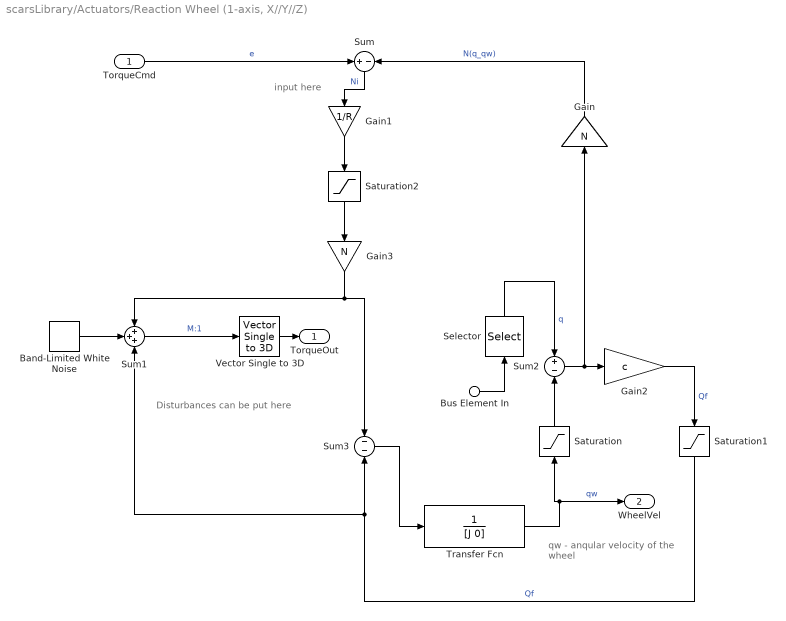
== system scarsLibrary/Actuators/Reaction Wheel (1-axis, X//Y//Z) ==
  note: qw - anqular velocity
      |  of the wheel
  note: input here
  note: Disturbances can
      | be put here
  TorqueCmd : Inport
  Bus Element In : Inport  Port=2  PortName=SatStates  Element=Omega_B
  Band-Limited White Noise : simulink/Sources/Band-Limited White Noise  Cov=rw_power  Ts=rw_freq  seed=[23341]
  Gain : Gain  Gain=N
  Gain1 : Gain  Gain=1/R
  Gain2 : Gain  Gain=c
  Gain3 : Gain  Gain=N
  Saturation : Saturate  UpperLimit=vel_max  LowerLimit=-vel_max
  Saturation1 : Saturate  UpperLimit=torq_max  LowerLimit=-torq_max
  Saturation2 : Saturate  UpperLimit=i_max  LowerLimit=-i_max
  Selector : Selector  InputPortWidth=3  IndexOptions=Index vector (dialog)  Indices=axis_switch  OutputSizes=1
  Sum : Sum  Inputs=+|-
  Sum1 : Sum  Inputs=+++
  Sum2 : Sum  Inputs=+|-
  Sum3 : Sum  Inputs=-|-
  Transfer Fcn : TransferFcn  Denominator=[J 0]
  "Vector Single to 3D " : $bdroot/Actuators/Vector Single to 3D   axis_switch=axis_switch
  TorqueOut : Outport
  WheelVel : Outport  Port=2
  wires:
  Selector/1 -> Sum2/1  "q"
  Gain/1 -> Sum/2  "N(q_qw)"
  Sum2/1 -> Gain/1, Gain2/1
  Sum1/1 -> "Vector Single to 3D "/1  "M:1"
  Saturation1/1 -> Sum1/3, Sum3/2  "Qf"
  Transfer Fcn/1 -> Saturation/1, WheelVel/1  "qw"
  Sum3/1 -> Transfer Fcn/1
  TorqueCmd/1 -> Sum/1  "e"
  Sum/1 -> Gain1/1  "Ni"
  Bus Element In/1 -> Selector/1
  "Vector Single to 3D "/1 -> TorqueOut/1
  Band-Limited White Noise/1 -> Sum1/2
  Saturation/1 -> Sum2/2
  Gain2/1 -> Saturation1/1  "Qf"
  Gain1/1 -> Saturation2/1
  Gain3/1 -> Sum1/1, Sum3/1
  Saturation2/1 -> Gain3/1

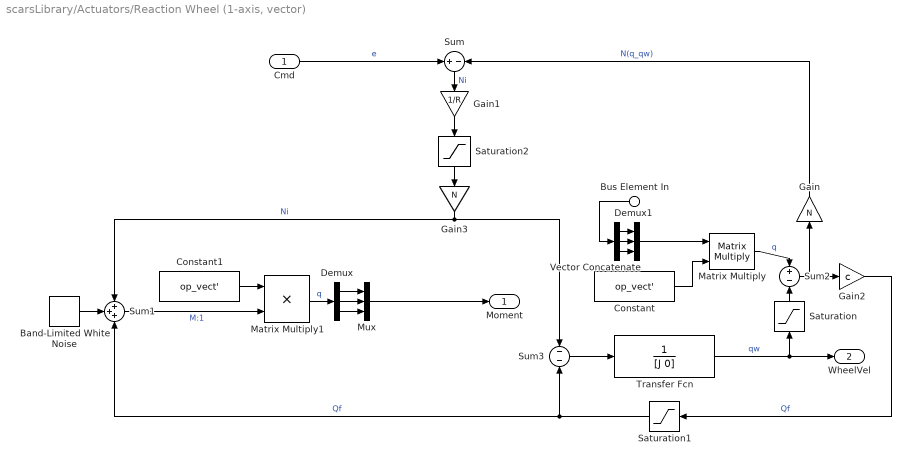
== system scarsLibrary/Actuators/Reaction Wheel (1-axis, vector) ==
  Cmd : Inport
  Bus Element In : Inport  Port=2  PortName=SatStates  Element=Omega_B
  Band-Limited White Noise : simulink/Sources/Band-Limited White Noise  Cov=rw_power  Ts=rw_freq  seed=[23341]
  Constant : Constant  Value=op_vect'  VectorParams1D=off
  Constant1 : Constant  Value=op_vect'  VectorParams1D=off
  Demux : Demux  Outputs=3
  Demux1 : Demux  Outputs=3
  Gain : Gain  Gain=N
  Gain1 : Gain  Gain=1/R
  Gain2 : Gain  Gain=c
  Gain3 : Gain  Gain=N
  Matrix Multiply : Product  Multiplication=Matrix(*)
  Matrix Multiply1 : Product
  Mux : Mux  Inputs=3
  Saturation : Saturate  UpperLimit=vel_max  LowerLimit=-vel_max
  Saturation1 : Saturate  UpperLimit=torq_max  LowerLimit=-torq_max
  Saturation2 : Saturate  UpperLimit=i_max  LowerLimit=-i_max
  Sum : Sum  Inputs=+|-
  Sum1 : Sum  Inputs=+++
  Sum2 : Sum  Inputs=+|-
  Sum3 : Sum  Inputs=-|-
  Transfer Fcn : TransferFcn  Denominator=[J 0]
  Vector Concatenate : Concatenate  NumInputs=3
  Moment : Outport
  WheelVel : Outport  Port=2
  wires:
  Gain1/1 -> Saturation2/1
  Saturation2/1 -> Gain3/1
  Sum3/1 -> Transfer Fcn/1
  Saturation1/1 -> Sum1/3, Sum3/2  "Qf"
  Transfer Fcn/1 -> Saturation/1, WheelVel/1  "qw"
  Gain/1 -> Sum/2  "N(q_qw)"
  Demux/3 -> Mux/3
  Demux/1 -> Mux/1
  Sum/1 -> Gain1/1  "Ni"
  Band-Limited White Noise/1 -> Sum1/2
  Matrix Multiply/1 -> Sum2/1  "q"
  Demux1/2 -> Vector Concatenate/2
  Vector Concatenate/1 -> Matrix Multiply/1
  Constant1/1 -> Matrix Multiply1/1
  Sum1/1 -> Matrix Multiply1/2  "M:1"
  Demux/2 -> Mux/2
  Constant/1 -> Matrix Multiply/2
  Matrix Multiply1/1 -> Demux/1  "q"
  Mux/1 -> Moment/1
  Sum2/1 -> Gain2/1, Gain/1
  Gain3/1 -> Sum3/1, Sum1/1  "Ni"
  Gain2/1 -> Saturation1/1  "Qf"
  Saturation/1 -> Sum2/2
  Demux1/3 -> Vector Concatenate/3
  Bus Element In/1 -> Demux1/1
  Cmd/1 -> Sum/1  "e"
  Demux1/1 -> Vector Concatenate/1

== system scarsLibrary/Actuators/Reaction Wheels ==
  TorqueCmd : Inport
  Bus Element In : Inport  Port=2  PortName=InBus  Element=Euler_NED
  Demux : Demux  Outputs=3
  Demux2 : Demux  Outputs=3
  Mux : Mux  Inputs=3
  Reaction Wheel Pitch : Subsystem
  Reaction Wheel Roll : Subsystem
  Reaction Wheel Yaw : Subsystem
  Torque : Outport  VectorParamsAs1DForOutWhenUnconnected=off
  wires:
  TorqueCmd/1 -> Demux/1
  Bus Element In/1 -> Demux2/1
  Reaction Wheel Yaw/1(Torque Out) -> Mux/3
  Reaction Wheel Pitch/1(Torque Out) -> Mux/2
  Demux/3 -> Reaction Wheel Yaw/2(Torque)
  Demux2/3 -> Reaction Wheel Yaw/1(Rate)
  Demux/2 -> Reaction Wheel Pitch/2(Torque)
  Demux2/2 -> Reaction Wheel Pitch/1(Rate)
  Demux2/1 -> Reaction Wheel Roll/1(Rate)
  Reaction Wheel Roll/1(Torque Out) -> Mux/1
  Demux/1 -> Reaction Wheel Roll/2(Torque)
  Mux/1 -> Torque/1

== system scarsLibrary/Actuators/Thruster ==
  ForceCmd : Inport
  Constant : Constant  Value=displacement
  Gain2 : Gain  Gain=-1
  Noise : simulink/Sources/Band-Limited White Noise  Cov=[0.1]  Ts=0.1  seed=[23341]
  Product : Product
  Relay1 : Relay  OnSwitchValue=bb.a1  OffSwitchValue=bb.a0  OnOutputValue=bb.thrust
  Relay2 : Relay  OnSwitchValue=bb.a1  OffSwitchValue=bb.a0  OnOutputValue=-bb.thrust
  Sum2 : Sum  Inputs=+++
  Transport Delay : TransportDelay  DelayTime=delay
  Force : Outport
  Moment : Outport  Port=2
  wires:
  ForceCmd/1 -> Transport Delay/1
  Relay1/1 -> Sum2/1
  Transport Delay/1 -> Gain2/1, Relay1/1
  Gain2/1 -> Relay2/1
  Noise/1 -> Sum2/2
  Sum2/1 -> Force/1
  Relay2/1 -> Product/1, Sum2/3
  Constant/1 -> Product/2
  Product/1 -> Moment/1

== system scarsLibrary/Environment/Atmosphere [kg//m^3] ==
  Bus Element In : Inport  PortName=SatStates  Element=lla
  Clock : Clock
      settings: Decimation=100
  Clock to Y/D/s : Subsystem
  "NRLMSISE-00 Atmosphere Model " : aerolibatmos2/NRLMSISE-00 Atmosphere Model  units=Metric (MKS)  lst_input=off  flux_ap_input=off  flags_input=Internal  flags=ones(1,23)  oxygen_in=off  action=Warning
      settings: SourceProductName=Aerospace Blockset  SourceProductBaseCode=AE
  "Selector " : Selector  InputPortWidth=9  IndexOptions=Index vector (dialog)  Indices=6  OutputSizes=1
  Terminator : Terminator
  Density : Outport
  wires:
  Clock to Y/D/s/1(Year) -> "NRLMSISE-00 Atmosphere Model "/2
  Clock to Y/D/s/3(sec) -> "NRLMSISE-00 Atmosphere Model "/4
  "Selector "/1 -> Density/1
  Bus Element In/1 -> "NRLMSISE-00 Atmosphere Model "/1
  Clock/1 -> Clock to Y/D/s/1(Clock)
  Clock to Y/D/s/2(Day) -> "NRLMSISE-00 Atmosphere Model "/3
  "NRLMSISE-00 Atmosphere Model "/1 -> Terminator/1
  "NRLMSISE-00 Atmosphere Model "/2 -> "Selector "/1

== system scarsLibrary/Environment/Atmospheric Drag [N] ==
  SatStates : Inport
  Atmosphere [kg/m^3] : $bdroot/Environment/Atmosphere [kg//m^3]  SystemSampleTime=-1  Latency=0  AutoFrameSizeCalculation=off
  Drag [N] : $bdroot/Environment/Drag [N]  SystemSampleTime=-1  Latency=0  AutoFrameSizeCalculation=off
  Force : Outport
  wires:
  Atmosphere [kg/m^3]/1 -> Drag [N]/2
  SatStates/1 -> Drag [N]/1, Atmosphere [kg/m^3]/1
  Drag [N]/1 -> Force/1

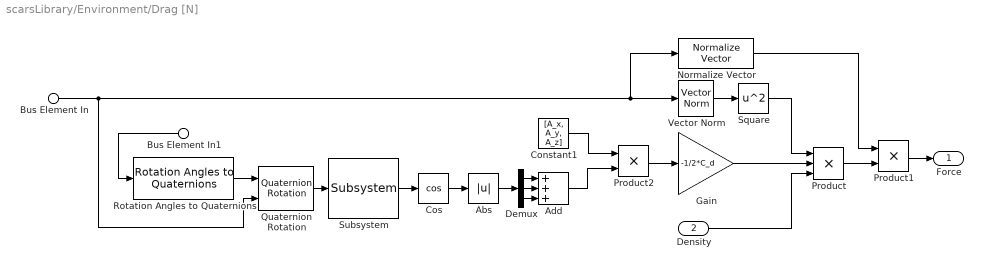
== system scarsLibrary/Environment/Drag [N] ==
  Bus Element In : Inport  PortName=SatStates  Element=V_B
  Bus Element In1 : Inport  PortName=SatStates  Element=Euler_B
  Density : Inport  Port=2
  Abs : Abs
  Add : Sum  Inputs=+++
  Constant1 : Constant  Value=[A_x, A_y, A_z]
  Cos : Trigonometry  Operator=cos
  Demux : Demux  Outputs=3
  Gain : Gain  Gain=-1/2*C_d
  Normalize Vector : vrlib/Utilities/Normalize Vector  maxzero=0
      settings: SourceProductName=Simulink
  Product : Product  Inputs=3
  Product1 : Product
  Product2 : Product
  Quaternion Rotation : aerolibutil/Quaternion Rotation
  Rotation Angles to Quaternions : sharedtransform/Rotation Angles to Quaternions  rotationOrder=XYZ  aMode=aMode
      settings: SourceProductName=Aerospace Blockset  SourceProductBaseCode=AE
  Square : Math  Operator=square  SignedPower=off  SaturateOnIntegerOverflow=on
  Subsystem : $bdroot/Subsystem  SystemSampleTime=-1  Latency=0  AutoFrameSizeCalculation=off
  Vector Norm : $bdroot/Vector Norm  SystemSampleTime=-1  Latency=0  AutoFrameSizeCalculation=off
  Force : Outport
  wires:
  Gain/1 -> Product/2
  Product/1 -> Product1/2
  Product1/1 -> Force/1
  Normalize Vector/1 -> Product1/1
  Density/1 -> Product/3
  Bus Element In1/1 -> Rotation Angles to Quaternions/1
  Constant1/1 -> Product2/1
  Product2/1 -> Gain/1
  Rotation Angles to Quaternions/1 -> Quaternion Rotation/1
  Bus Element In/1 -> Vector Norm/1, Normalize Vector/1, Quaternion Rotation/2
  Quaternion Rotation/1 -> Subsystem/1
  Subsystem/1 -> Cos/1
  Demux/1 -> Add/1
  Demux/2 -> Add/2
  Demux/3 -> Add/3
  Cos/1 -> Abs/1
  Add/1 -> Product2/2
  Vector Norm/1 -> Square/1
  Square/1 -> Product/1
  Abs/1 -> Demux/1

== system scarsLibrary/Environment/Environment ==
  SatStates : Inport
  Atmosphere [kg/m^3] : $bdroot/Environment/Atmosphere [kg//m^3]  SystemSampleTime=-1  Latency=0  AutoFrameSizeCalculation=off
  Atmospheric Drag [N] : $bdroot/Environment/Atmospheric Drag [N]  SystemSampleTime=-1  Latency=0  AutoFrameSizeCalculation=off
      link override Drag [N]/Constant1: Value=area_vector
  Bus Creator : BusCreator  Inputs=4
  Bus Selector : BusSelector  OutputSignals=DCM_ECEF2B
  Gravity [N] : $bdroot/Environment/Gravity [N]  mass=0
  Ground : Ground
  Invert 3x3 Matrix : aerolibutil/Invert  3x3 Matrix
  Magnetic Field [nT] : $bdroot/Environment/Magnetic Field [nT]  SystemSampleTime=-1  Latency=0  AutoFrameSizeCalculation=off
  Matrix Multiply : Product  Multiplication=Matrix(*)
  Sum : Sum  Inputs=+|+
  Sun's Position [km] : $bdroot/Environment/Sun's Position [km]  SystemSampleTime=-1  Latency=0  AutoFrameSizeCalculation=off
  Forces : Outport
  Moments : Outport  Port=2
  Env : Outport  Port=3
  wires:
  SatStates/1 -> Magnetic Field [nT]/1, Gravity [N]/1, Bus Selector/1, Atmospheric Drag [N]/1, Atmosphere [kg/m^3]/1
  Sum/1 -> Bus Creator/2, Forces/1  "Environment Force [N]"
  Sun's Position [km]/1 -> Bus Creator/3  "Sun's Position [km]"
  Magnetic Field [nT]/1 -> Bus Creator/1  "Magnetic Field [nT]"
  Gravity [N]/1 -> Sum/1
  Bus Creator/1 -> Env/1
  Atmosphere [kg/m^3]/1 -> Bus Creator/4  "Atmosphere Density [kg/m^3]"
  Ground/1 -> Moments/1
  Atmospheric Drag [N]/1 -> Matrix Multiply/2
  Invert 3x3 Matrix/1 -> Matrix Multiply/1
  Bus Selector/1 -> Invert 3x3 Matrix/1  "<DCM_ECEF2B>"
  Matrix Multiply/1 -> Sum/2

== system scarsLibrary/Environment/Gravity [N] ==
  Bus Element In : Inport  PortName=SatStates  Element=X_ECEF
  Gain : Gain  Gain=mass
  Spherical Harmonic Gravity Model1 : aerolibgravity2/Spherical Harmonic Gravity Model  units=Metric (MKS)  degree=120  action=Warning  ptype=EGM2008  datafile='aerogmm2b.mat'
      settings: SourceProductName=Aerospace Blockset  SourceProductBaseCode=AE
  To Workspace13 : ToWorkspace  VariableName=g  SampleTime=-1
  Force : Outport
  wires:
  Spherical Harmonic Gravity Model1/1 -> To Workspace13/1, Gain/1
  Bus Element In/1 -> Spherical Harmonic Gravity Model1/1
  Gain/1 -> Force/1

== system scarsLibrary/Environment/Magnetic Field [nT] ==
  SatStates : Inport
  Clock : Clock
  Magnetic Model : Subsystem
  Time2Decyear : Subsystem
  B : Outport
  wires:
  Clock/1 -> Time2Decyear/1(" ")
  Time2Decyear/1("  ") -> Magnetic Model/1(DecimalYear)
  SatStates/1 -> Magnetic Model/2(SatStates)
  Magnetic Model/1(MagneticField) -> B/1

== system scarsLibrary/Environment/Sun's Position [km] ==
  1-D Lookup Table : Lookup_n-D  NumberOfTableDimensions=1  BreakpointsForDimension1=sun_position(:,1)  Table=sun_position(:,2)  InternalRulePriority=Speed  RndMeth=Simplest  InputSameDT=on
  1-D Lookup Table1 : Lookup_n-D  NumberOfTableDimensions=1  BreakpointsForDimension1=sun_position(:,1)  Table=sun_position(:,3)  InternalRulePriority=Speed  RndMeth=Simplest  InputSameDT=on
  1-D Lookup Table2 : Lookup_n-D  NumberOfTableDimensions=1  BreakpointsForDimension1=sun_position(:,1)  Table=sun_position(:,4)  InternalRulePriority=Speed  RndMeth=Simplest  InputSameDT=on
  Clock : Clock
  Mux : Mux  Inputs=3
  X_ecef : Outport
  wires:
  1-D Lookup Table1/1 -> Mux/2
  1-D Lookup Table2/1 -> Mux/3
  Clock/1 -> 1-D Lookup Table/1, 1-D Lookup Table2/1, 1-D Lookup Table1/1
  Mux/1 -> X_ecef/1  "Sun's Position [km]"
  1-D Lookup Table/1 -> Mux/1  "Sun's Position [km]"

== system scarsLibrary/Other/Actuator Noise ==
  In : Inport
  Constant : Constant  Value=added_noise
  Gain : Gain  Gain=1+multiplied_noise
  Sum : Sum  Inputs=|++
  Out : Outport
  wires:
  Sum/1 -> Out/1
  In/1 -> Gain/1
  Constant/1 -> Sum/2
  Gain/1 -> Sum/1

== system scarsLibrary/Other/Subsystem ==
  Vector : Inport
  Atan1 : Trigonometry  Operator=atan2
  Atan2 : Trigonometry  Operator=atan2
  Atan3 : Trigonometry  Operator=atan2
  Mux : Mux  Inputs=3
  Selector : Selector  InputPortWidth=3  IndexOptions=Index vector (dialog)  Indices=[1 2]  OutputSizes=1
  Selector1 : Selector  InputPortWidth=3  IndexOptions=Index vector (dialog)  Indices=[2 3]  OutputSizes=1
  Selector2 : Selector  InputPortWidth=3  IndexOptions=Index vector (dialog)  Indices=[1 3]  OutputSizes=1
  Selector3 : Selector  InputPortWidth=3  IndexOptions=Index vector (dialog)  Indices=2  OutputSizes=1
  Selector4 : Selector  InputPortWidth=3  IndexOptions=Index vector (dialog)  Indices=1  OutputSizes=1
  Selector5 : Selector  InputPortWidth=3  IndexOptions=Index vector (dialog)  Indices=3  OutputSizes=1
  Vector Norm : $bdroot/Vector Norm  SystemSampleTime=-1  Latency=0  AutoFrameSizeCalculation=off
  Vector Norm1 : $bdroot/Vector Norm  SystemSampleTime=-1  Latency=0  AutoFrameSizeCalculation=off
  Vector Norm2 : $bdroot/Vector Norm  SystemSampleTime=-1  Latency=0  AutoFrameSizeCalculation=off
  Angles : Outport
  wires:
  Selector5/1 -> Atan3/2
  Vector/1 -> Selector1/1, Selector4/1, Selector2/1, Selector5/1, Selector/1, Selector3/1
  Selector4/1 -> Atan1/2
  Mux/1 -> Angles/1
  Selector1/1 -> Vector Norm/1
  Selector3/1 -> Atan2/2
  Vector Norm2/1 -> Atan3/1
  Vector Norm1/1 -> Atan2/1
  Vector Norm/1 -> Atan1/1
  Atan1/1 -> Mux/1
  Atan2/1 -> Mux/2
  Atan3/1 -> Mux/3
  Selector/1 -> Vector Norm2/1
  Selector2/1 -> Vector Norm1/1

== system scarsLibrary/Other/Subsystem1 ==
  SatStates : Inport
  Bus Selector : BusSelector  OutputSignals=V_ECEF,X_ECEF
  <V_ECEF> : Outport
  <X_ECEF> : Outport  Port=2
  wires:
  SatStates/1 -> Bus Selector/1
  Bus Selector/1 -> <V_ECEF>/1  "<V_ECEF>"
  Bus Selector/2 -> <X_ECEF>/1  "<X_ECEF>"

== system scarsLibrary/Other/Subsystem4 ==
  Angle : Inport
  Cos2 : Trigonometry  Operator=cos
  Cos3 : Trigonometry  Operator=cos
  Demux : Demux  Outputs=3
  Mux1 : Mux  Inputs=3
  Product : Product
  Product1 : Product
  Sin : Trigonometry
  Sin1 : Trigonometry
  Terminator : Terminator
  Vector : Outport
  wires:
  Product/1 -> Mux1/1
  Cos3/1 -> Product/2
  Sin1/1 -> Product1/2
  Demux/2 -> Cos2/1, Sin/1
  Angle/1 -> Demux/1
  Demux/3 -> Cos3/1, Sin1/1
  Cos2/1 -> Product1/1, Product/1
  Mux1/1 -> Vector/1
  Demux/1 -> Terminator/1
  Sin/1 -> Mux1/3
  Product1/1 -> Mux1/2

== system scarsLibrary/Other/Unit Pulse ==
  Step : Step  Time=startTime  SampleTime=0
  Step1 : Step  Time=startTime+length  After=-1  SampleTime=0
  Sum : Sum  Inputs=|++
  " Pulse" : Outport
  wires:
  Sum/1 -> " Pulse"/1
  Step1/1 -> Sum/2
  Step/1 -> Sum/1

== system scarsLibrary/Other/Unit Pulse Product ==
  In : Inport
  Product : Product
  Step : Step  Time=startTime  SampleTime=0
  Step1 : Step  Time=startTime+length  After=-1  SampleTime=0
  Sum : Sum  Inputs=|++
  " Pulse" : Outport
  wires:
  Step/1 -> Sum/1
  Sum/1 -> Product/1
  Step1/1 -> Sum/2
  In/1 -> Product/2
  Product/1 -> " Pulse"/1

== system scarsLibrary/Other/Vector Norm ==
  In : Inport
  Dot Product : DotProduct  InputSameDT=on  OutDataTypeStr=Inherit: Inherit via internal rule
  Sqrt : Sqrt  SaturateOnIntegerOverflow=on
  Out : Outport
  wires:
  Sqrt/1 -> Out/1
  Dot Product/1 -> Sqrt/1
  In/1 -> Dot Product/1, Dot Product/2

== system scarsLibrary/Other/Vector Single to 3D  ==
  In : Inport
  Constant : Constant  Value=axis_switch
  Ground{,1..5} (6 alike) : Ground
  Multiport Switch : MultiPortSwitch
  Mux : Mux  Inputs=3
  Mux1 : Mux  Inputs=3
  Mux2 : Mux  Inputs=3
  Out : Outport
  wires:
  Ground5/1 -> Mux2/3
  Constant/1 -> Multiport Switch/1
  In/1 -> Mux2/2, Mux/3, Mux1/1
  Ground3/1 -> Mux1/3
  Ground2/1 -> Mux1/2
  Mux1/1 -> Multiport Switch/2
  Mux2/1 -> Multiport Switch/3
  Mux/1 -> Multiport Switch/4
  Ground1/1 -> Mux/1
  Ground/1 -> Mux/2
  Ground4/1 -> Mux2/1
  Multiport Switch/1 -> Out/1

== system scarsLibrary/PW-Sat2/Drag Sail ==
  SatStates : Inport
  Bus Element In : Inport  Port=2  PortName=Env  Element=Atmosphere Density [kg/m^3]
  Add : Sum
  Deployment Duration : Step  Time=ds_time+ds_duration  After=-1  SampleTime=0
  Deployment Time : Step  Time=ds_time  SampleTime=0
  Depoloyment Moments : Constant  Value=ds_moments
  "Drag " : Subsystem
  Gain : Gain
  Product : Product
  Product1 : Product
  Product3 : Product
  Force : Outport
  Moment : Outport  Port=2
  wires:
  Gain/1 -> Force/1
  Product3/1 -> Add/2
  Product1/1 -> Add/1
  Deployment Duration/1 -> Product3/2
  Depoloyment Moments/1 -> Product3/1, Product1/2
  Add/1 -> Moment/1
  "Drag "/1(Force) -> Product/1
  Deployment Time/1 -> Product/2, Product1/1
  SatStates/1 -> "Drag "/1(SatStates)
  Product/1 -> Gain/1
  Bus Element In/1 -> "Drag "/2(Density)
